simulink model "TestADCTrippleMode"  (R2015b)
settings: Solver=FixedStepDiscrete  StartTime=0.0  StopTime=10.0  FixedStep=0.5  RelTol=1e-3
libraries: ADC_Lib x3, USART_Lib x3, DAC_Lib x1, STM32_Config_Lib x1
settings Model: Creator=reynaudp  LastModifiedBy=reynaudp
settings DataIOCC: SaveFormat=Array  SignalLoggingSaveFormat=ModelDataLogs
settings OptimizationCC: OptimizeModelRefInitCode=on  LifeSpan=1
settings DebuggingCC: UnderspecifiedInitializationDetection=Classic  MergeDetectMultiDrivingBlocksExec=none  SolverPrmCheckMsg=warning  MultiTaskDSMMsg=warning  MultiTaskCondExecSysMsg=none
settings HardwareCC: ProdBitPerPointer=32  ProdLargestAtomicInteger=Integer  ProdWordSize=32  ProdHWDeviceType=STMicroelectronics->STM32 32-bit Cortex-M  TargetBitPerPointer=64  TargetLongLongMode=on  TargetIntDivRoundTo=Zero  TargetEndianess=LittleEndian  TargetWordSize=64  TargetHWDeviceType=MATLAB Host  ProdEqTarget=off
settings RTWCC: SystemTargetFile=stm32.tlc  TemplateMakefile=stm32.tmf  Description=stm32 (Embedded Target)  GenerateReport=on  IncludeHyperlinkInReport=on  LaunchReport=on
settings CodeAppCC: IgnoreCustomStorageClasses=off  MaxIdLength=64  CustomSymbolStrType=$N$R$M  SimulinkBlockComments=off
settings STFCustomTargetCC: CodeReplacementLibrary=ARM CMSIS SIN COS  ParMdlRefBuildCompliant=on  ConcurrentExecutionCompliant=off  IncludeMdlTerminateFcn=off  GeneratePreprocessorConditionals=Use local settings  CombineOutputUpdateFcns=on  ERTCustomFileBanners=on  SupportContinuousTime=off  SupportNonInlinedSFcns=off  MATLABClassNameForMDSCustomization=Simulink.SoftwareTarget.ERTCustomization  CPPClassGenCompliant=off  GRTInterface=off  SystemTargetFile=stm32.tlc
settings ERTTargetCC: CodeReplacementLibrary=ARM CMSIS SIN COS  CompOptLevelCompliant=off  ConcurrentExecutionCompliant=off  IncludeMdlTerminateFcn=off  ERTFirstTimeCompliant=off  ModelStepFunctionPrototypeControlCompliant=off  CPPClassGenCompliant=off  UseToolchainInfoCompliant=off  ERTSrcFileBannerTemplate=sourceFileTemplate.cgt  ERTHdrFileBannerTemplate=sourceFileTemplate.cgt  ERTDataSrcFileTemplate=sourceFileTemplate.cgt  ERTDataHdrFileTemplate=sourceFileTemplate.cgt  ERTCustomFileTemplate=customRoutineProcess.tlc
settings ConfigComp: CovModelRefEnable=Off  CovSFcnEnable=off

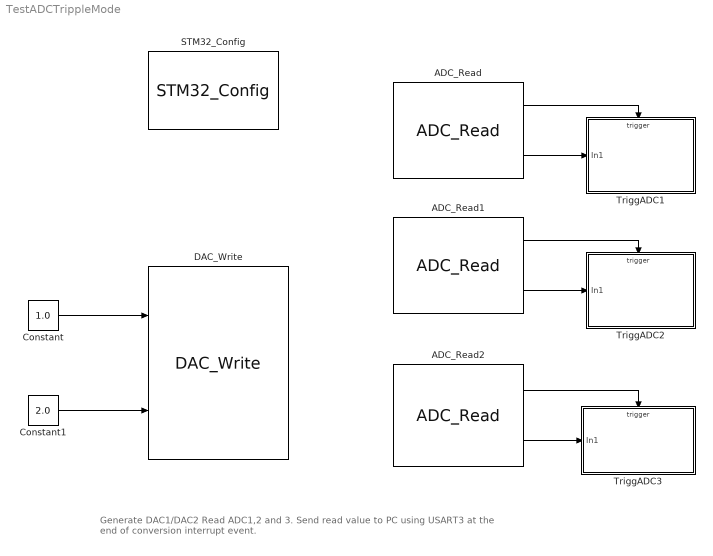
== system TestADCTrippleMode ==
  note: Generate DAC1/DAC2
      | Read ADC1,2 and 3.
      | Send read value to PC using USART3 at the end of conversion interrupt event.
  ADC_Read : ADC_Lib/ADC_Read  ADC_Name=ADC1  ADC_Ch0=off  ADC_Ch1=on  ADC_Ch2=off  ADC_Ch3=off  ADC_Ch4=off  ADC_Ch5=off  ADC_Ch6=off  ADC_Ch7=off  ADC_Ch8=off  ADC_Ch9=off  ADC_Ch10=off  ADC_Ch11=off  ADC_Ch12=off  ADC_Ch13=off  ADC_Ch14=off  ADC_Ch15=off  ADC_Ch16=off  ADC_Ch17=off  ADC_Ch18=off  RgRk1=off  RgRk2=off  RgRk3=off  RgRk4=off  RgRk1_Ch=Ch0_r1  RgRk2_Ch=off  RgRk3_Ch=off  RgRk4_Ch=off  RgRk5=off  RgRk6=off  RgRk7=off  RgRk8=off  RgRk5_Ch=off  RgRk6_Ch=off  RgRk7_Ch=off  RgRk8_Ch=off  RgRk9=off  RgRk10=off  RgRk11=off  RgRk12=off  RgRk9_Ch=off  RgRk10_Ch=off  RgRk11_Ch=off  RgRk12_Ch=off  RgRk13=off  RgRk14=off  RgRk15=off  RgRk16=off  RgRk13_Ch=off  RgRk14_Ch=off  RgRk15_Ch=off  RgRk16_Ch=off  InjRk1=off  InjRk2=on  InjRk3=off  InjRk4=off  InjRk1_Ch=Ch0_i1  InjRk2_Ch=Ch1_i2  InjRk3_Ch=Ch2_i3  InjRk4_Ch=off  ADC_Trig=Not used  ADC_TrigEdge=Not used  DmaReq=on  ItReq=on  AWD_Mode=NOT_USED  AWD_Ch=0  AWD_HThres=0  AWD_LThres=0  AWD_En_Int=off  AWD2_HThres=0  AWD2_LThres=0  AWD2_En_Int=off  AWD3_HThres=0  AWD3_LThres=0  AWD3_En_Int=off  EOC_IT=on  JEOC_IT=off  AWD_IT=off  OVR_IT=off  ADC_RegNb=1  ADC_RegCh0=on  ADC_RegCh1=off  ADC_RegCh2=off  ADC_RegCh3=off  ADC_RegCh4=off  ADC_RegCh5=off  ADC_RegCh6=off  ADC_RegCh7=off  ADC_RegCh8=off  ADC_RegCh9=off  ADC_RegCh10=off  ADC_RegCh11=off  ADC_RegCh12=off  ADC_RegCh13=off  ADC_RegCh14=off  ADC_RegCh15=off  ADC_RegCh16=off  ADC_RegCh17=off  ADC_RegCh18=off  ADC_InjNb=3  ADC_InjCh0=on  ADC_InjCh1=on  ADC_InjCh2=on  ADC_InjCh3=off  ADC_InjCh4=off  ADC_InjCh5=off  ADC_InjCh6=off  ADC_InjCh7=off  ADC_InjCh8=off  ADC_InjCh9=off  ADC_InjCh10=off  ADC_InjCh11=off  ADC_InjCh12=off  ADC_InjCh13=off  ADC_InjCh14=off  ADC_InjCh15=off  ADC_InjCh16=off  ADC_InjCh17=off  ADC_InjCh18=off  ADC_RegRank0=1  ADC_RegRank1=0  ADC_RegRank2=0  ADC_RegRank3=0  ADC_RegRank4=0  ADC_RegRank5=0  ADC_RegRank6=0  ADC_RegRank7=0  ADC_RegRank8=0  ADC_RegRank9=0  ADC_RegRank10=0  ADC_RegRank11=0  ADC_RegRank12=0  ADC_RegRank13=0  ADC_RegRank14=0  ADC_RegRank15=0  ADC_RegRank16=0  ADC_RegRank17=0  ADC_RegRank18=0  ADC_InjRank0=1  ADC_InjRank1=2  ADC_InjRank2=3  ADC_InjRank3=0  ADC_InjRank4=0  ADC_InjRank5=0  ADC_InjRank6=0  ADC_InjRank7=0  ADC_InjRank8=0  ADC_InjRank9=0  ADC_InjRank10=0  ADC_InjRank11=0  ADC_InjRank12=0  ADC_InjRank13=0  ADC_InjRank14=0  ADC_InjRank15=0  ADC_InjRank16=0  ADC_InjRank17=0  ADC_InjRank18=0  NbADC=3  CurrentADC=ADC1
  ADC_Read1 : ADC_Lib/ADC_Read  ADC_Name=ADC2  ADC_Ch0=off  ADC_Ch1=off  ADC_Ch2=off  ADC_Ch3=on  ADC_Ch4=off  ADC_Ch5=off  ADC_Ch6=off  ADC_Ch7=off  ADC_Ch8=off  ADC_Ch9=off  ADC_Ch10=off  ADC_Ch11=off  ADC_Ch12=off  ADC_Ch13=off  ADC_Ch14=off  ADC_Ch15=off  ADC_Ch16=off  ADC_Ch17=off  ADC_Ch18=off  RgRk1=on  RgRk2=off  RgRk3=off  RgRk4=off  RgRk1_Ch=Ch3_r1  RgRk2_Ch=off  RgRk3_Ch=off  RgRk4_Ch=off  RgRk5=off  RgRk6=off  RgRk7=off  RgRk8=off  RgRk5_Ch=off  RgRk6_Ch=off  RgRk7_Ch=off  RgRk8_Ch=off  RgRk9=off  RgRk10=off  RgRk11=off  RgRk12=off  RgRk9_Ch=off  RgRk10_Ch=off  RgRk11_Ch=off  RgRk12_Ch=off  RgRk13=off  RgRk14=off  RgRk15=off  RgRk16=off  RgRk13_Ch=off  RgRk14_Ch=off  RgRk15_Ch=off  RgRk16_Ch=off  InjRk1=off  InjRk2=off  InjRk3=off  InjRk4=off  InjRk1_Ch=Ch3_i1  InjRk2_Ch=Ch6_i2  InjRk3_Ch=Ch7_i3  InjRk4_Ch=off  ADC_Trig=Not used  ADC_TrigEdge=Not used  DmaReq=on  ItReq=on  AWD_Mode=NOT_USED  AWD_Ch=0  AWD_HThres=0  AWD_LThres=0  AWD_En_Int=off  AWD2_HThres=0  AWD2_LThres=0  AWD2_En_Int=off  AWD3_HThres=0  AWD3_LThres=0  AWD3_En_Int=off  EOC_IT=on  JEOC_IT=off  AWD_IT=off  OVR_IT=off  ADC_RegNb=1  ADC_RegCh0=off  ADC_RegCh1=off  ADC_RegCh2=off  ADC_RegCh3=on  ADC_RegCh4=off  ADC_RegCh5=off  ADC_RegCh6=off  ADC_RegCh7=off  ADC_RegCh8=off  ADC_RegCh9=off  ADC_RegCh10=off  ADC_RegCh11=off  ADC_RegCh12=off  ADC_RegCh13=off  ADC_RegCh14=off  ADC_RegCh15=off  ADC_RegCh16=off  ADC_RegCh17=off  ADC_RegCh18=off  ADC_InjNb=3  ADC_InjCh0=off  ADC_InjCh1=off  ADC_InjCh2=off  ADC_InjCh3=on  ADC_InjCh4=off  ADC_InjCh5=off  ADC_InjCh6=on  ADC_InjCh7=on  ADC_InjCh8=off  ADC_InjCh9=off  ADC_InjCh10=off  ADC_InjCh11=off  ADC_InjCh12=off  ADC_InjCh13=off  ADC_InjCh14=off  ADC_InjCh15=off  ADC_InjCh16=off  ADC_InjCh17=off  ADC_InjCh18=off  ADC_RegRank0=0  ADC_RegRank1=0  ADC_RegRank2=0  ADC_RegRank3=1  ADC_RegRank4=0  ADC_RegRank5=0  ADC_RegRank6=0  ADC_RegRank7=0  ADC_RegRank8=0  ADC_RegRank9=0  ADC_RegRank10=0  ADC_RegRank11=0  ADC_RegRank12=0  ADC_RegRank13=0  ADC_RegRank14=0  ADC_RegRank15=0  ADC_RegRank16=0  ADC_RegRank17=0  ADC_RegRank18=0  ADC_InjRank0=0  ADC_InjRank1=0  ADC_InjRank2=0  ADC_InjRank3=1  ADC_InjRank4=0  ADC_InjRank5=0  ADC_InjRank6=2  ADC_InjRank7=3  ADC_InjRank8=0  ADC_InjRank9=0  ADC_InjRank10=0  ADC_InjRank11=0  ADC_InjRank12=0  ADC_InjRank13=0  ADC_InjRank14=0  ADC_InjRank15=0  ADC_InjRank16=0  ADC_InjRank17=0  ADC_InjRank18=0  NbADC=3  CurrentADC=ADC2
  ADC_Read2 : ADC_Lib/ADC_Read  ADC_Name=ADC3  ADC_Ch0=off  ADC_Ch1=off  ADC_Ch2=off  ADC_Ch3=off  ADC_Ch4=off  ADC_Ch5=off  ADC_Ch6=off  ADC_Ch7=off  ADC_Ch8=off  ADC_Ch9=off  ADC_Ch10=off  ADC_Ch11=off  ADC_Ch12=off  ADC_Ch13=on  ADC_Ch14=off  ADC_Ch15=off  ADC_Ch16=off  ADC_Ch17=off  ADC_Ch18=off  RgRk1=off  RgRk2=off  RgRk3=off  RgRk4=off  RgRk1_Ch=Ch12_r1  RgRk2_Ch=off  RgRk3_Ch=off  RgRk4_Ch=off  RgRk5=off  RgRk6=off  RgRk7=off  RgRk8=off  RgRk5_Ch=off  RgRk6_Ch=off  RgRk7_Ch=off  RgRk8_Ch=off  RgRk9=off  RgRk10=off  RgRk11=off  RgRk12=off  RgRk9_Ch=off  RgRk10_Ch=off  RgRk11_Ch=off  RgRk12_Ch=off  RgRk13=off  RgRk14=off  RgRk15=off  RgRk16=off  RgRk13_Ch=off  RgRk14_Ch=off  RgRk15_Ch=off  RgRk16_Ch=off  InjRk1=off  InjRk2=on  InjRk3=off  InjRk4=off  InjRk1_Ch=Ch12_i1  InjRk2_Ch=Ch13_i2  InjRk3_Ch=Ch12_i3  InjRk4_Ch=off  ADC_Trig=Not used  ADC_TrigEdge=Not used  DmaReq=on  ItReq=on  AWD_Mode=NOT_USED  AWD_Ch=0  AWD_HThres=0  AWD_LThres=0  AWD_En_Int=off  AWD2_HThres=0  AWD2_LThres=0  AWD2_En_Int=off  AWD3_HThres=0  AWD3_LThres=0  AWD3_En_Int=off  EOC_IT=on  JEOC_IT=off  AWD_IT=off  OVR_IT=off  ADC_RegNb=1  ADC_RegCh0=off  ADC_RegCh1=off  ADC_RegCh2=off  ADC_RegCh3=off  ADC_RegCh4=off  ADC_RegCh5=off  ADC_RegCh6=off  ADC_RegCh7=off  ADC_RegCh8=off  ADC_RegCh9=off  ADC_RegCh10=off  ADC_RegCh11=off  ADC_RegCh12=on  ADC_RegCh13=off  ADC_RegCh14=off  ADC_RegCh15=off  ADC_RegCh16=off  ADC_RegCh17=off  ADC_RegCh18=off  ADC_InjNb=3  ADC_InjCh0=off  ADC_InjCh1=off  ADC_InjCh2=off  ADC_InjCh3=off  ADC_InjCh4=off  ADC_InjCh5=off  ADC_InjCh6=off  ADC_InjCh7=off  ADC_InjCh8=off  ADC_InjCh9=off  ADC_InjCh10=off  ADC_InjCh11=off  ADC_InjCh12=on  ADC_InjCh13=on  ADC_InjCh14=off  ADC_InjCh15=off  ADC_InjCh16=off  ADC_InjCh17=off  ADC_InjCh18=off  ADC_RegRank0=0  ADC_RegRank1=0  ADC_RegRank2=0  ADC_RegRank3=0  ADC_RegRank4=0  ADC_RegRank5=0  ADC_RegRank6=0  ADC_RegRank7=0  ADC_RegRank8=0  ADC_RegRank9=0  ADC_RegRank10=0  ADC_RegRank11=0  ADC_RegRank12=1  ADC_RegRank13=0  ADC_RegRank14=0  ADC_RegRank15=0  ADC_RegRank16=0  ADC_RegRank17=0  ADC_RegRank18=0  ADC_InjRank0=0  ADC_InjRank1=0  ADC_InjRank2=0  ADC_InjRank3=0  ADC_InjRank4=0  ADC_InjRank5=0  ADC_InjRank6=0  ADC_InjRank7=0  ADC_InjRank8=0  ADC_InjRank9=0  ADC_InjRank10=0  ADC_InjRank11=0  ADC_InjRank12=3  ADC_InjRank13=2  ADC_InjRank14=0  ADC_InjRank15=0  ADC_InjRank16=0  ADC_InjRank17=0  ADC_InjRank18=0  NbADC=3  CurrentADC=ADC3
  Constant : Constant  Value=1.0  OutDataTypeStr=double
  Constant1 : Constant  Value=2.0  OutDataTypeStr=double
  DAC_Write : DAC_Lib/DAC_Write  Pin0=on  Pin1=on  PinList="DAC0  1"
  STM32_Config : STM32_Config_Lib/STM32_Config  Priority=0  Project_Path=.\  Config_File=TestADCTrippleMode.ioc  MCU_Name=STM32F407VGTx
  TriggADC1 : Subsystem  TreatAsAtomicUnit=on
  TriggADC2 : Subsystem  TreatAsAtomicUnit=on
  TriggADC3 : Subsystem  TreatAsAtomicUnit=on
  wires:
  ADC_Read1/1 -> TriggADC2/Trigger
  Constant/1 -> DAC_Write/1
  Constant1/1 -> DAC_Write/2
  ADC_Read/2 -> TriggADC1/1(In1)
  ADC_Read/1 -> TriggADC1/Trigger
  ADC_Read1/2 -> TriggADC2/1(In1)
  ADC_Read2/1 -> TriggADC3/Trigger
  ADC_Read2/2 -> TriggADC3/1(In1)

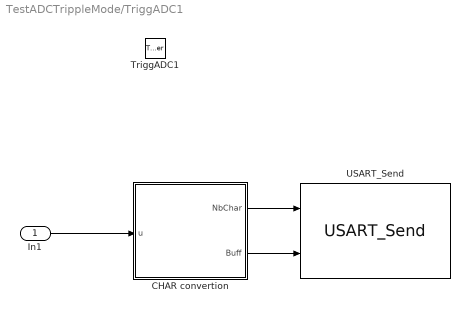
== system TestADCTrippleMode/TriggADC1 ==
  In1 : Inport
  TriggADC1 : TriggerPort  TriggerType=function-call
  CHAR convertion : MATLAB Function  TreatAsAtomicUnit=on
  USART_Send : USART_Lib/USART_Send  USART_name=USART3  Buff_size=512  nbUsart=1  usartMode=Asynchronous  usartDma_Rx=off  usartDma_Tx=off  usartIt=on
  wires:
  CHAR convertion/1(NbChar) -> USART_Send/1
  CHAR convertion/2(Buff) -> USART_Send/2
  In1/1 -> CHAR convertion/1(u)

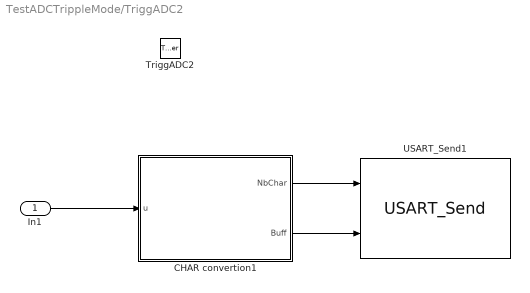
== system TestADCTrippleMode/TriggADC2 ==
  In1 : Inport
  TriggADC2 : TriggerPort  TriggerType=function-call
  CHAR convertion1 : MATLAB Function  TreatAsAtomicUnit=on
  USART_Send1 : USART_Lib/USART_Send  USART_name=USART3  Buff_size=512  nbUsart=1  usartMode=Asynchronous  usartDma_Rx=off  usartDma_Tx=off  usartIt=on
  wires:
  CHAR convertion1/1(NbChar) -> USART_Send1/1
  CHAR convertion1/2(Buff) -> USART_Send1/2
  In1/1 -> CHAR convertion1/1(u)

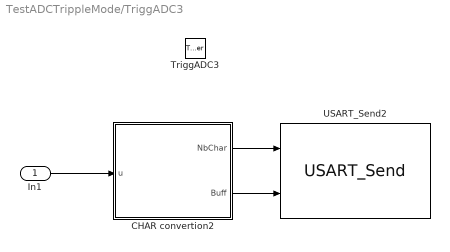
== system TestADCTrippleMode/TriggADC3 ==
  In1 : Inport
  TriggADC3 : TriggerPort  TriggerType=function-call
  CHAR convertion2 : MATLAB Function  TreatAsAtomicUnit=on
  USART_Send2 : USART_Lib/USART_Send  USART_name=USART3  Buff_size=512  nbUsart=1  usartMode=Asynchronous  usartDma_Rx=off  usartDma_Tx=off  usartIt=on
  wires:
  CHAR convertion2/2(Buff) -> USART_Send2/2
  In1/1 -> CHAR convertion2/1(u)
  CHAR convertion2/1(NbChar) -> USART_Send2/1

== matlab function TestADCTrippleMode/TriggADC2/CHAR convertion1 ==
  data: u input; NbChar output uint16 size=1; Buff output uint32 size=1
function [NbChar, Buff] = convert(u)
if coder.target('Sfun')
% Executing in MATLAB, Buff is null
Buff = uint32(0);
NbChar = uint16(0);
else
% Executing in the generated code. 
buffer = zeros(1,15,'uint8');
strLen = int32(0);
strLen = coder.ceval('sprintf',coder.wref(buffer),['%2.2f',0],u);
%tmp = buffer(1:strLen);
tmp = uint8('(B)');
y = [buffer(1:4), tmp, 13, 10, 0];
%Buff = uint32(coder.ref(y));
Buff = coder.ceval('getBuffPtr',coder.ref(y));
NbChar = uint16(size(y,2));
end
end
%Buff = uint32(y);
%%Buff = [buffer(1:4), tmp, 13, 10, 0];

== matlab function TestADCTrippleMode/TriggADC1/CHAR convertion ==
  data: u input; NbChar output uint16 size=1; Buff output uint32 size=1
function [NbChar, Buff] = convert(u)
if coder.target('Sfun')
% Executing in MATLAB, Buff is null
Buff = uint32(0);
NbChar = uint16(0);
else
% Executing in the generated code. 
buffer = zeros(1,15,'uint8');
strLen = int32(0);
strLen = coder.ceval('sprintf',coder.wref(buffer),['%2.2f',0],u);
%tmp = buffer(1:strLen);
tmp = uint8('(A)');
y = [buffer(1:4), tmp, 13, 10, 0];
%Buff = uint32(coder.ref(y));
Buff = coder.ceval('getBuffPtr',coder.ref(y));
NbChar = uint16(size(y,2));
end
end
%Buff = uint32(y);
%%Buff = [buffer(1:4), tmp, 13, 10, 0];

== matlab function TestADCTrippleMode/TriggADC3/CHAR convertion2 ==
  data: u input; NbChar output uint16 size=1; Buff output uint32 size=1
function [NbChar, Buff] = convert(u)
if coder.target('Sfun')
% Executing in MATLAB, Buff is null
Buff = uint32(0);
NbChar = uint16(0);
else
% Executing in the generated code. 
buffer = zeros(1,15,'uint8');
strLen = int32(0);
strLen = coder.ceval('sprintf',coder.wref(buffer),['%2.2f',0],u);
%tmp = buffer(1:strLen);
tmp = uint8('(C)');
y = [buffer(1:4), tmp, 13, 10, 0];
%Buff = uint32(coder.ref(y));
Buff = coder.ceval('getBuffPtr',coder.ref(y));
NbChar = uint16(size(y,2));
end
end
%Buff = uint32(y);
%%Buff = [buffer(1:4), tmp, 13, 10, 0];
